simulink model "ADRClibriry"  (R2018a)
settings: Solver=VariableStepAuto  StartTime=0.0  StopTime=10.0  RelTol=1e-3
undefined symbols (not defined in the file or in its folder): sigbuilder_block
libraries: simulink x7, dspswit3 x4
(part 2 of 2)

== system ADRClibriry/ADRC_controller_NLSEF/roll_ADRC1 ==
  States : Inport  OutDataTypeStr=Bus: StatesBus
  <roll_cmd> : Inport  Port=2
  u_x : Inport  Port=3
  Bus Selector1 : BusSelector  OutputSignals=Euler
  ESO : Demux  Outputs=3
  Gain2 : Gain  Gain=0.025504
  Gain3 : Gain  Gain=39.2418
  MATLAB Function : MATLAB Function  TreatAsAtomicUnit=on
  Mux : Mux  Inputs=2
  RT : RateTransition  OutPortSampleTime=0.05
  RT1 : RateTransition  OutPortSampleTime=0.01
  S-Function : S-Function  FunctionName=s_TD  SFunctionDeploymentMode=off  EnableBusSupport=off
  S-Function4 : S-Function  FunctionName=s_ESO  SFunctionDeploymentMode=off  EnableBusSupport=off
  Scope : Scope  NumInputPorts=2
  Scope1 : Scope
  Scope2 : Scope  NumInputPorts=2
  Scope4 : Scope  NumInputPorts=2
  Sine Wave : Sin  Amplitude=0.2  Frequency=2*pi*1  Phase=2*pi*1.5  SampleTime=0.01
  TD : Demux  Outputs=2
  Terminator : Terminator
  Terminator1 : Terminator
  angle : Demux  Outputs=3
  "u_p " : Outport
  d_1 : Outport  Port=2
  wires:
  Mux/1 -> S-Function4/1
  States/1 -> Bus Selector1/1
  Gain3/1 -> Mux/2
  ESO/3 -> Gain2/1
  <roll_cmd>/1 -> RT/1, Scope/1
  angle/1 -> Scope2/2, Mux/1
  Bus Selector1/1 -> angle/1  "<Euler>"
  RT/1 -> S-Function/1
  S-Function4/1 -> ESO/1
  RT1/1 -> TD/1
  TD/2 -> MATLAB Function/2(x2_d), Scope1/1
  Gain2/1 -> d_1/1
  S-Function/1 -> RT1/1
  TD/1 -> MATLAB Function/1(x1_d), Scope/2
  angle/3 -> Terminator1/1
  angle/2 -> Terminator/1
  ESO/2 -> MATLAB Function/4(x2)
  MATLAB Function/1(y) -> "u_p "/1
  Sine Wave/1 -> Scope4/1
  ESO/1 -> MATLAB Function/3(x1), Scope2/1
  u_x/1 -> Gain3/1

== system ADRClibriry/ADRC_controller_NLSEF/yaw_ADRC ==
  States : Inport  OutDataTypeStr=Bus: StatesBus
  <yaw_cmd> : Inport  Port=2
  Add : Sum  Inputs=+-
  Bus Selector1 : BusSelector  OutputSignals=Euler
  Demux : Demux  Outputs=2
  ESO : Demux  Outputs=3
  Gain2 : Gain  Gain=0.00562
  Gain3 : Gain  Gain=1/0.00562
  MATLAB Function : MATLAB Function  TreatAsAtomicUnit=on
  Manual Switch : ManualSwitch  CurrentSetting=0
  Mux : Mux  Inputs=2
  RT : RateTransition
  RT1 : RateTransition
  S-Function : S-Function  FunctionName=s_yawTD  SFunctionDeploymentMode=off  EnableBusSupport=off
  S-Function4 : S-Function  FunctionName=s_ESO  SFunctionDeploymentMode=off  EnableBusSupport=off
  Scope{,1..2,4} (4 alike) : Scope  NumInputPorts=2
  Scope3 : Scope
  Sine Wave : Sin  Amplitude=0.05  Frequency=2*pi*1  SampleTime=0.01
  Terminator : Terminator
  Terminator1 : Terminator
  angle : Demux  Outputs=3
  u_r : Outport
  wires:
  Mux/1 -> S-Function4/1
  States/1 -> Bus Selector1/1
  ESO/1 -> Scope4/2, MATLAB Function/3(x1), Scope1/1
  Gain3/1 -> Mux/2
  ESO/3 -> Gain2/1
  <yaw_cmd>/1 -> Manual Switch/2, Scope/2
  ESO/2 -> MATLAB Function/4(x2)
  Bus Selector1/1 -> angle/1  "<Euler>"
  RT/1 -> S-Function/1
  S-Function4/1 -> ESO/1
  Add/1 -> Scope3/1, u_r/1, Gain3/1
  RT1/1 -> Demux/1
  Demux/2 -> Scope2/1, MATLAB Function/2(x2_d)
  Gain2/1 -> Add/2
  S-Function/1 -> RT1/1
  Demux/1 -> MATLAB Function/1(x1_d), Scope/1
  angle/3 -> Scope1/2, Mux/1
  angle/2 -> Terminator1/1
  angle/1 -> Terminator/1
  MATLAB Function/1(y) -> Add/1
  Sine Wave/1 -> Manual Switch/1, Scope4/1
  Manual Switch/1 -> RT/1

== system ADRClibriry/ADRC_controller_NLSEF1/Subsystem ==
  In1 : Inport
  In2 : Inport  Port=2
  In3 : Inport  Port=3
  Divide : Product  Inputs=*/
  Gain : Gain  Gain=-1225^2/9.788
  Product : Product
  Saturation1 : Saturate  UpperLimit=1  LowerLimit=0.5
  Sqrt : Sqrt  SaturateOnIntegerOverflow=on
  Trigonometric Function : Trigonometry  Operator=cos
  Trigonometric Function1 : Trigonometry  Operator=cos
  speed : Outport
  wires:
  Saturation1/1 -> Divide/2
  Trigonometric Function/1 -> Product/1
  In3/1 -> Divide/1
  Trigonometric Function1/1 -> Product/2
  In2/1 -> Trigonometric Function/1
  Product/1 -> Saturation1/1
  In1/1 -> Trigonometric Function1/1
  Divide/1 -> Gain/1
  Gain/1 -> Sqrt/1
  Sqrt/1 -> speed/1

== system ADRClibriry/ADRC_controller_NLSEF1/Subsystem2 ==
  u_1 : Inport
  u_2 : Inport  Port=2
  u_3 : Inport  Port=3
  u_4 : Inport  Port=4
  u_5 : Inport  Port=5
  d_3 : Inport  Port=6
  Demux3 : Demux  Outputs=7
  Mux : Mux  Inputs=6
  S-Function1 : S-Function  FunctionName=s_Optim1  SFunctionDeploymentMode=off  EnableBusSupport=off
  Saturation{1..4} (4 alike) : Saturate  UpperLimit=0.3491  LowerLimit=-0.3491
  c1 : Outport
  c2 : Outport  Port=2
  c3 : Outport  Port=3
  c4 : Outport  Port=4
  ux : Outport  Port=5
  uy : Outport  Port=6
  uz : Outport  Port=7
  wires:
  Demux3/4 -> Saturation4/1
  Saturation3/1 -> c3/1  "c3"
  u_3/1 -> Mux/3
  u_1/1 -> Mux/1
  Saturation1/1 -> c1/1  "c1"
  Demux3/1 -> Saturation1/1
  Saturation4/1 -> c4/1  "c4"
  Demux3/2 -> Saturation2/1
  u_2/1 -> Mux/2
  Saturation2/1 -> c2/1  "c2"
  Demux3/3 -> Saturation3/1
  Mux/1 -> S-Function1/1
  S-Function1/1 -> Demux3/1
  u_4/1 -> Mux/4
  d_3/1 -> Mux/6
  u_5/1 -> Mux/5
  Demux3/5 -> ux/1
  Demux3/6 -> uy/1
  Demux3/7 -> uz/1

== system ADRClibriry/ADRC_controller_NLSEF1/Subsystem3 ==
  u_p : Inport
  u_q : Inport  Port=2
  u_r : Inport  Port=3
  p : Inport  Port=4
  q : Inport  Port=5
  speed : Inport  Port=6
  Add1 : Sum
  Add2 : Sum  Inputs=+-
  Add3 : Sum  Inputs=+-
  Constant1 : Constant  Value=0.000029
  Constant2 : Constant  Value=0.04238
  Product{,1..3} (4 alike) : Product
  u_1 : Outport
  u_2 : Outport  Port=2
  u_3 : Outport  Port=3
  wires:
  Add3/1 -> u_3/1
  Add1/1 -> u_1/1
  Constant1/1 -> Product1/1, Product/2
  q/1 -> Product/1
  Product1/1 -> Product2/1
  Constant2/1 -> Add3/2
  u_p/1 -> Add1/2
  p/1 -> Product1/2
  Add2/1 -> u_2/1
  Product3/1 -> Add1/1
  speed/1 -> Product3/2, Product2/2
  Product/1 -> Product3/1
  Product2/1 -> Add2/2
  u_q/1 -> Add2/1
  u_r/1 -> Add3/1

== system ADRClibriry/ADRC_controller_NLSEF1/h_ADRC ==
  note: 控制器输出为升力提供的加速度
  States : Inport  OutDataTypeStr=Bus: StatesBus
  <throttle_cmd> : Inport  Port=2
  Add : Sum  Inputs=+-
  Bus Selector1 : BusSelector  OutputSignals=X_ned
  Constant : Constant  Value=9.78
  Demux : Demux  Outputs=2
  ESO : Demux  Outputs=3
  Gain2 : Gain
  Gain3 : Gain
  MATLAB Function : MATLAB Function  TreatAsAtomicUnit=on
  Mux : Mux  Inputs=2
  RT : RateTransition  OutPortSampleTime=0.05
  RT1 : RateTransition  OutPortSampleTime=0.01
  S-Function : S-Function  FunctionName=s_TD  SFunctionDeploymentMode=off  EnableBusSupport=off
  S-Function4 : S-Function  FunctionName=s_ESO  SFunctionDeploymentMode=off  EnableBusSupport=off
  Scope3 : Scope
  Sum2 : Sum  Inputs=++|
  Sum3 : Sum  Inputs=|++
  Terminator : Terminator
  Terminator1 : Terminator
  x : Demux  Outputs=3
  a_t : Outport
  wires:
  Mux/1 -> S-Function4/1
  States/1 -> Bus Selector1/1
  ESO/1 -> MATLAB Function/3(x1)
  Gain3/1 -> Sum2/2
  ESO/3 -> Sum3/1
  <throttle_cmd>/1 -> RT/1
  ESO/2 -> MATLAB Function/4(x2)
  Bus Selector1/1 -> x/1  "<X_ned>"
  RT/1 -> S-Function/1
  S-Function4/1 -> ESO/1
  RT1/1 -> Demux/1
  Demux/2 -> MATLAB Function/2(x2_d)
  Gain2/1 -> Add/2, Scope3/1
  S-Function/1 -> RT1/1
  Demux/1 -> MATLAB Function/1(x1_d)
  x/3 -> Mux/1
  x/2 -> Terminator/1
  x/1 -> Terminator1/1
  Add/1 -> a_t/1, Gain3/1  "a_t"
  Sum2/1 -> Mux/2
  Sum3/1 -> Gain2/1
  Constant/1 -> Sum3/2, Sum2/1
  MATLAB Function/1(y) -> Add/1

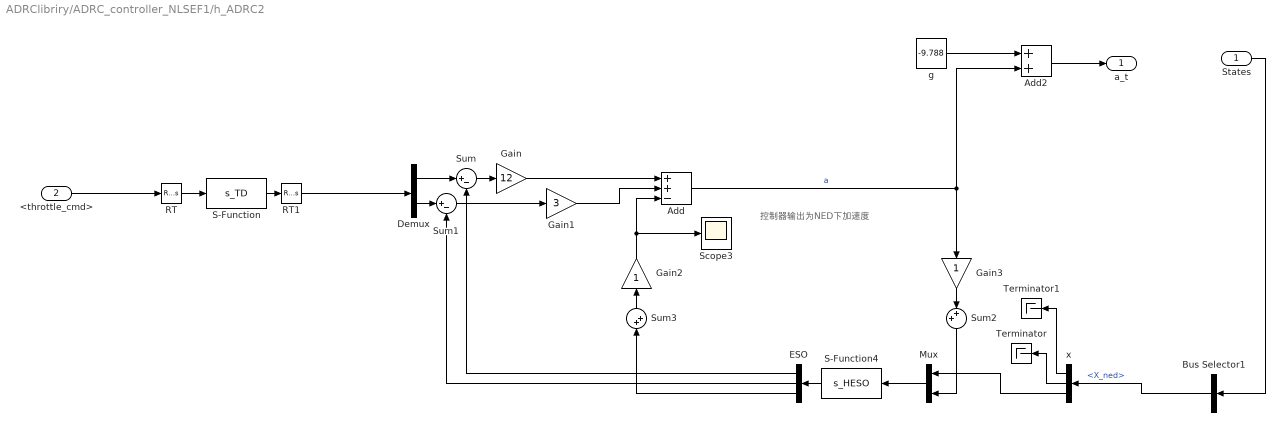
== system ADRClibriry/ADRC_controller_NLSEF1/h_ADRC2 ==
  note: 控制器输出为NED下加速度
  States : Inport  OutDataTypeStr=Bus: StatesBus
  <throttle_cmd> : Inport  Port=2
  Add : Sum  Inputs=++-
  Add2 : Sum
  Bus Selector1 : BusSelector  OutputSignals=X_ned
  Demux : Demux  Outputs=2
  ESO : Demux  Outputs=3
  Gain : Gain  Gain=12
  Gain1 : Gain  Gain=3
  Gain2 : Gain
  Gain3 : Gain
  Mux : Mux  Inputs=2
  RT : RateTransition  OutPortSampleTime=0.05
  RT1 : RateTransition  OutPortSampleTime=0.01
  S-Function : S-Function  FunctionName=s_TD  SFunctionDeploymentMode=off  EnableBusSupport=off
  S-Function4 : S-Function  FunctionName=s_HESO  SFunctionDeploymentMode=off  EnableBusSupport=off
  Scope3 : Scope
  Sum : Sum  Inputs=|+-
  Sum1 : Sum  Inputs=|+-
  Sum2 : Sum  Inputs=++|
  Sum3 : Sum  Inputs=|++
  Terminator : Terminator
  Terminator1 : Terminator
  g : Constant  Value=-9.788
  x : Demux  Outputs=3
  a_t : Outport
  wires:
  Gain1/1 -> Add/2
  Mux/1 -> S-Function4/1
  States/1 -> Bus Selector1/1
  ESO/1 -> Sum/2
  Gain3/1 -> Sum2/2
  ESO/3 -> Sum3/1
  <throttle_cmd>/1 -> RT/1
  ESO/2 -> Sum1/2
  Bus Selector1/1 -> x/1  "<X_ned>"
  RT/1 -> S-Function/1
  S-Function4/1 -> ESO/1
  Sum1/1 -> Gain1/1
  Gain/1 -> Add/1
  RT1/1 -> Demux/1
  Demux/2 -> Sum1/1
  Gain2/1 -> Add/3, Scope3/1
  S-Function/1 -> RT1/1
  Sum/1 -> Gain/1
  Demux/1 -> Sum/1
  x/3 -> Mux/1
  x/2 -> Terminator/1
  x/1 -> Terminator1/1
  Add/1 -> Add2/2, Gain3/1  "a"
  Sum2/1 -> Mux/2
  Sum3/1 -> Gain2/1
  Add2/1 -> a_t/1
  g/1 -> Add2/1

== system ADRClibriry/ADRC_controller_NLSEF1/h_ADRC3 ==
  note: 控制器输出为升力
  States : Inport  OutDataTypeStr=Bus: StatesBus
  <throttle_cmd> : Inport  Port=2
  Add : Sum  Inputs=++-
  Bus Selector1 : BusSelector  OutputSignals=X_ned
  Constant : Constant  Value=9.78
  Demux : Demux  Outputs=2
  ESO : Demux  Outputs=3
  Gain : Gain  Gain=12
  Gain1 : Gain  Gain=3
  Gain2 : Gain  Gain=1.53
  Gain3 : Gain  Gain=1/1.53
  Gain4 : Gain  Gain=1/1.53
  Mux : Mux  Inputs=2
  RT : RateTransition  OutPortSampleTime=0.05
  RT1 : RateTransition  OutPortSampleTime=0.01
  S-Function : S-Function  FunctionName=s_TD  SFunctionDeploymentMode=off  EnableBusSupport=off
  S-Function4 : S-Function  FunctionName=s_HESO  SFunctionDeploymentMode=off  EnableBusSupport=off
  Sum : Sum  Inputs=|+-
  Sum1 : Sum  Inputs=|+-
  Sum2 : Sum  Inputs=++|
  Sum3 : Sum  Inputs=|++
  Terminator : Terminator
  Terminator1 : Terminator
  x : Demux  Outputs=3
  a_t : Outport
  wires:
  Gain1/1 -> Add/2
  Mux/1 -> S-Function4/1
  States/1 -> Bus Selector1/1
  ESO/1 -> Sum/2
  Gain3/1 -> Sum2/2
  ESO/3 -> Sum3/1
  <throttle_cmd>/1 -> RT/1
  ESO/2 -> Sum1/2
  Bus Selector1/1 -> x/1  "<X_ned>"
  RT/1 -> S-Function/1
  S-Function4/1 -> ESO/1
  Sum1/1 -> Gain1/1
  Gain/1 -> Add/1
  RT1/1 -> Demux/1
  Demux/2 -> Sum1/1
  Gain2/1 -> Add/3
  S-Function/1 -> RT1/1
  Sum/1 -> Gain/1
  Demux/1 -> Sum/1
  x/3 -> Mux/1
  x/2 -> Terminator/1
  x/1 -> Terminator1/1
  Add/1 -> Gain4/1, Gain3/1  "T"
  Sum2/1 -> Mux/2
  Sum3/1 -> Gain2/1
  Constant/1 -> Sum3/2, Sum2/1
  Gain4/1 -> a_t/1

== system ADRClibriry/ADRC_controller_NLSEF1/pitch_ADRC ==
  States : Inport  OutDataTypeStr=Bus: StatesBus
  <pitch_cmd> : Inport  Port=2
  u_y : Inport  Port=3
  Add : Sum  Inputs=+-
  Bus Selector1 : BusSelector  OutputSignals=Euler
  Demux : Demux  Outputs=2
  ESO : Demux  Outputs=3
  Gain : Gain  Gain=0.025504
  Gain5 : Gain  Gain=39.2418
  MATLAB Function : MATLAB Function  TreatAsAtomicUnit=on
  Mux : Mux  Inputs=2
  RT : RateTransition  OutPortSampleTime=0.05
  RT1 : RateTransition  OutPortSampleTime=0.01
  S-Function : S-Function  FunctionName=s_TD  SFunctionDeploymentMode=off  EnableBusSupport=off
  S-Function4 : S-Function  FunctionName=s_ESO  SFunctionDeploymentMode=off  EnableBusSupport=off
  Scope4 : Scope  NumInputPorts=2
  Sine Wave : Sin  Amplitude=0.2  Frequency=2*pi*1  SampleTime=0.01
  Terminator : Terminator
  Terminator1 : Terminator
  angle : Demux  Outputs=3
  "u_q " : Outport
  wires:
  Mux/1 -> S-Function4/1
  States/1 -> Bus Selector1/1
  Gain5/1 -> Mux/2
  ESO/3 -> Gain/1
  Bus Selector1/1 -> angle/1  "<Euler>"
  RT/1 -> S-Function/1
  S-Function4/1 -> ESO/1
  RT1/1 -> Demux/1
  Demux/2 -> MATLAB Function/2(x2_d)
  S-Function/1 -> RT1/1
  angle/3 -> Terminator1/1
  angle/2 -> Mux/1
  ESO/2 -> MATLAB Function/4(x2)
  Demux/1 -> MATLAB Function/1(x1_d)
  <pitch_cmd>/1 -> RT/1
  angle/1 -> Terminator/1
  ESO/1 -> MATLAB Function/3(x1)
  Sine Wave/1 -> Scope4/1
  MATLAB Function/1(y) -> Add/1
  Add/1 -> "u_q "/1
  u_y/1 -> Gain5/1
  Gain/1 -> Add/2

== system ADRClibriry/ADRC_controller_NLSEF1/roll_ADRC ==
  States : Inport  OutDataTypeStr=Bus: StatesBus
  <roll_cmd> : Inport  Port=2
  u_x : Inport  Port=3
  Add : Sum  Inputs=+-
  Bus Selector1 : BusSelector  OutputSignals=Euler
  ESO : Demux  Outputs=3
  Gain2 : Gain  Gain=0.025504
  Gain3 : Gain  Gain=39.2418
  MATLAB Function : MATLAB Function  TreatAsAtomicUnit=on
  Mux : Mux  Inputs=2
  RT : RateTransition  OutPortSampleTime=0.05
  RT1 : RateTransition  OutPortSampleTime=0.01
  S-Function : S-Function  FunctionName=s_TD  SFunctionDeploymentMode=off  EnableBusSupport=off
  S-Function4 : S-Function  FunctionName=s_ESO  SFunctionDeploymentMode=off  EnableBusSupport=off
  Scope : Scope  NumInputPorts=2
  Scope1 : Scope
  Scope2 : Scope  NumInputPorts=2
  Scope4 : Scope  NumInputPorts=2
  Sine Wave : Sin  Amplitude=0.2  Frequency=2*pi*1  Phase=2*pi*1.5  SampleTime=0.01
  TD : Demux  Outputs=2
  Terminator : Terminator
  Terminator1 : Terminator
  angle : Demux  Outputs=3
  "u_p " : Outport
  wires:
  RT/1 -> S-Function/1
  ESO/3 -> Gain2/1
  S-Function4/1 -> ESO/1
  RT1/1 -> TD/1
  angle/2 -> Terminator/1
  Gain2/1 -> Add/2
  MATLAB Function/1(y) -> Add/1
  angle/1 -> Scope2/2, Mux/1
  Bus Selector1/1 -> angle/1  "<Euler>"
  Sine Wave/1 -> Scope4/1
  TD/2 -> MATLAB Function/2(x2_d), Scope1/1
  ESO/2 -> MATLAB Function/4(x2)
  Gain3/1 -> Mux/2
  S-Function/1 -> RT1/1
  ESO/1 -> MATLAB Function/3(x1), Scope2/1
  States/1 -> Bus Selector1/1
  Mux/1 -> S-Function4/1
  TD/1 -> MATLAB Function/1(x1_d), Scope/2
  u_x/1 -> Gain3/1
  angle/3 -> Terminator1/1
  <roll_cmd>/1 -> RT/1, Scope/1
  Add/1 -> "u_p "/1

== system ADRClibriry/ADRC_controller_NLSEF1/roll_ADRC1 ==
  States : Inport  OutDataTypeStr=Bus: StatesBus
  <roll_cmd> : Inport  Port=2
  u_x : Inport  Port=3
  Bus Selector1 : BusSelector  OutputSignals=Euler
  ESO : Demux  Outputs=3
  Gain2 : Gain  Gain=0.025504
  Gain3 : Gain  Gain=39.2418
  MATLAB Function : MATLAB Function  TreatAsAtomicUnit=on
  Mux : Mux  Inputs=2
  RT : RateTransition  OutPortSampleTime=0.05
  RT1 : RateTransition  OutPortSampleTime=0.01
  S-Function : S-Function  FunctionName=s_TD  SFunctionDeploymentMode=off  EnableBusSupport=off
  S-Function4 : S-Function  FunctionName=s_ESO  SFunctionDeploymentMode=off  EnableBusSupport=off
  Scope : Scope  NumInputPorts=2
  Scope1 : Scope
  Scope2 : Scope  NumInputPorts=2
  Scope4 : Scope  NumInputPorts=2
  Sine Wave : Sin  Amplitude=0.2  Frequency=2*pi*1  Phase=2*pi*1.5  SampleTime=0.01
  TD : Demux  Outputs=2
  Terminator : Terminator
  Terminator1 : Terminator
  angle : Demux  Outputs=3
  "u_p " : Outport
  d_1 : Outport  Port=2
  wires:
  Mux/1 -> S-Function4/1
  States/1 -> Bus Selector1/1
  Gain3/1 -> Mux/2
  ESO/3 -> Gain2/1
  <roll_cmd>/1 -> RT/1, Scope/1
  angle/1 -> Scope2/2, Mux/1
  Bus Selector1/1 -> angle/1  "<Euler>"
  RT/1 -> S-Function/1
  S-Function4/1 -> ESO/1
  RT1/1 -> TD/1
  TD/2 -> MATLAB Function/2(x2_d), Scope1/1
  Gain2/1 -> d_1/1
  S-Function/1 -> RT1/1
  TD/1 -> MATLAB Function/1(x1_d), Scope/2
  angle/3 -> Terminator1/1
  angle/2 -> Terminator/1
  ESO/2 -> MATLAB Function/4(x2)
  MATLAB Function/1(y) -> "u_p "/1
  Sine Wave/1 -> Scope4/1
  ESO/1 -> MATLAB Function/3(x1), Scope2/1
  u_x/1 -> Gain3/1

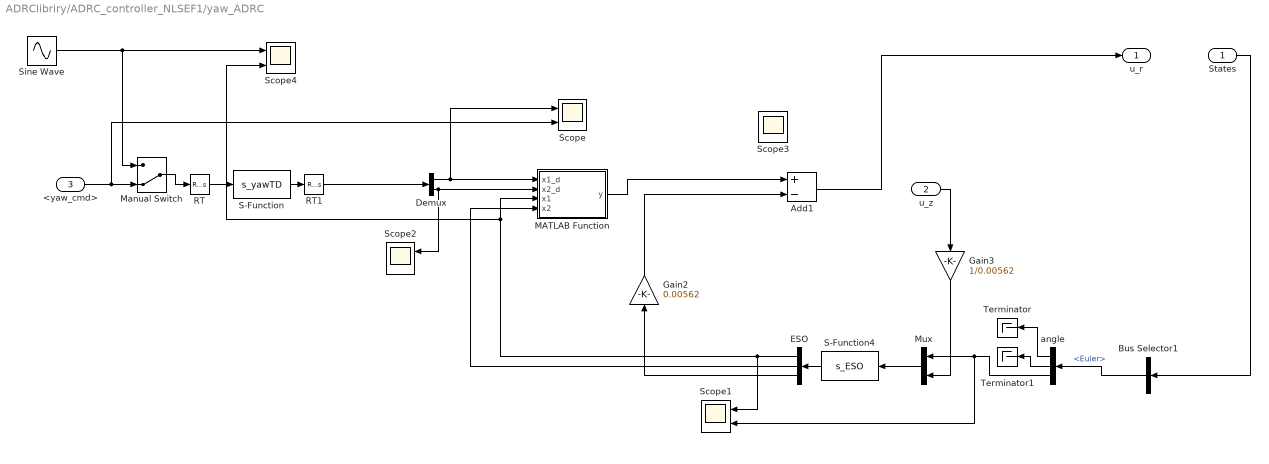
== system ADRClibriry/ADRC_controller_NLSEF1/yaw_ADRC ==
  States : Inport  OutDataTypeStr=Bus: StatesBus
  u_z : Inport  Port=2
  <yaw_cmd> : Inport  Port=3
  Add1 : Sum  Inputs=+-
  Bus Selector1 : BusSelector  OutputSignals=Euler
  Demux : Demux  Outputs=2
  ESO : Demux  Outputs=3
  Gain2 : Gain  Gain=0.00562
  Gain3 : Gain  Gain=1/0.00562
  MATLAB Function : MATLAB Function  TreatAsAtomicUnit=on
  Manual Switch : ManualSwitch  CurrentSetting=0
  Mux : Mux  Inputs=2
  RT : RateTransition
  RT1 : RateTransition
  S-Function : S-Function  FunctionName=s_yawTD  SFunctionDeploymentMode=off  EnableBusSupport=off
  S-Function4 : S-Function  FunctionName=s_ESO  SFunctionDeploymentMode=off  EnableBusSupport=off
  Scope{,1..2,4} (4 alike) : Scope  NumInputPorts=2
  Scope3 : Scope
  Sine Wave : Sin  Amplitude=0.05  Frequency=2*pi*1  SampleTime=0.01
  Terminator : Terminator
  Terminator1 : Terminator
  angle : Demux  Outputs=3
  u_r : Outport
  wires:
  Mux/1 -> S-Function4/1
  States/1 -> Bus Selector1/1
  ESO/1 -> Scope4/2, MATLAB Function/3(x1), Scope1/1
  Gain3/1 -> Mux/2
  ESO/3 -> Gain2/1
  <yaw_cmd>/1 -> Manual Switch/2, Scope/2
  ESO/2 -> MATLAB Function/4(x2)
  Bus Selector1/1 -> angle/1  "<Euler>"
  RT/1 -> S-Function/1
  S-Function4/1 -> ESO/1
  RT1/1 -> Demux/1
  Demux/2 -> Scope2/1, MATLAB Function/2(x2_d)
  S-Function/1 -> RT1/1
  Demux/1 -> MATLAB Function/1(x1_d), Scope/1
  angle/3 -> Scope1/2, Mux/1
  angle/2 -> Terminator1/1
  angle/1 -> Terminator/1
  Sine Wave/1 -> Manual Switch/1, Scope4/1
  Manual Switch/1 -> RT/1
  Gain2/1 -> Add1/2
  MATLAB Function/1(y) -> Add1/1
  Add1/1 -> u_r/1
  u_z/1 -> Gain3/1

== system ADRClibriry/PID_controller1/Signal Builder ==
  Demux : Demux  Tag=STV Demux
  FromWs : FromWorkspace  Tag=STV FromWs  VariableName=tuvar  SampleTime=0
      SigBuilderData=|
      | common.afterFinalStr = 'Extrapolate'
      | common.sampleTime = 0
      | dataSet.timeRange = [0 50]
      | dataSet.name = 'Group 1'
      | sbobj.Groups.Name = 'Group 1'
      | sbobj.Groups.Signals(1).Name = 'roll_cmd'
      | sbobj.Groups.Signals(1).XData = [0 6 6 8.55 8.55 10.7 10.7 13 13 50]
      | sbobj.Groups.Signals(1).YData = [0 0 0.05 0.05 0 0 -0.05 -0.05 0 0]
      | sbobj.Groups.Signals(2).Name = 'picth_cmd'
      | sbobj.Groups.Signals(2).XData = [0 14.9 14.9 17.5 17.5 20.8 50]
      | sbobj.Groups.Signals(2).YData = [0 0 0.05 0.05 0 0 0]
      | sbobj.Groups.Signals(3).Name = 'yaw_cmd'
      | sbobj.Groups.Signals(3).XData = [0 33.4 33.4 39.4 39.4 40.9 40.9 46.65 46.65 50]
      | sbobj.Groups.Signals(3).YData = [0 0 0.1 0.1 0 0 -0.1 -0.1 0 0]
      | sbobj.Groups.Signals(4).Name = 'throttle_cmd'
      | sbobj.Groups.Signals(4).XData = [0 10 21.35 21.35 26.15 32.4 50]
      | sbobj.Groups.Signals(4).YData = [0 -1.8 -1.8 -3.8 -3.8 -3.8 -3.8]
      | sbobj.Groups.TimeRange = [0 50]
  roll_cmd : Outport  Tag=STV Outport
  picth_cmd : Outport  Tag=STV Outport  Port=2
  yaw_cmd : Outport  Tag=STV Outport  Port=3
  throttle_cmd : Outport  Tag=STV Outport  Port=4
  wires:
  Demux/1 -> roll_cmd/1
  FromWs/1 -> Demux/1
  Demux/2 -> picth_cmd/1
  Demux/3 -> yaw_cmd/1
  Demux/4 -> throttle_cmd/1

== system ADRClibriry/PID_controller1/Subsystem ==
  In1 : Inport
  In2 : Inport  Port=2
  In3 : Inport  Port=3
  Divide : Product  Inputs=*/
  Gain : Gain  Gain=-1225^2/9.788
  Product : Product
  Saturation1 : Saturate  UpperLimit=1  LowerLimit=0.5
  Sqrt : Sqrt  SaturateOnIntegerOverflow=on
  Trigonometric Function : Trigonometry  Operator=cos
  Trigonometric Function1 : Trigonometry  Operator=cos
  speed : Outport
  wires:
  Saturation1/1 -> Divide/2
  Trigonometric Function/1 -> Product/1
  In3/1 -> Divide/1
  Trigonometric Function1/1 -> Product/2
  In2/1 -> Trigonometric Function/1
  Product/1 -> Saturation1/1
  In1/1 -> Trigonometric Function1/1
  Divide/1 -> Gain/1
  Gain/1 -> Sqrt/1
  Sqrt/1 -> speed/1

== system ADRClibriry/PID_controller1/Subsystem2 ==
  u_1 : Inport
  u_2 : Inport  Port=2
  u_3 : Inport  Port=3
  u_4 : Inport  Port=4
  u_5 : Inport  Port=5
  d_3 : Inport  Port=6
  Demux3 : Demux  Outputs=7
  Mux : Mux  Inputs=6
  S-Function1 : S-Function  FunctionName=s_Optim2  SFunctionDeploymentMode=off  EnableBusSupport=off
  Saturation{1..4} (4 alike) : Saturate  UpperLimit=0.3491  LowerLimit=-0.3491
  c1 : Outport
  c2 : Outport  Port=2
  c3 : Outport  Port=3
  c4 : Outport  Port=4
  ux : Outport  Port=5
  uy : Outport  Port=6
  uz : Outport  Port=7
  wires:
  Demux3/4 -> Saturation4/1
  Saturation3/1 -> c3/1  "c3"
  u_3/1 -> Mux/3
  u_1/1 -> Mux/1
  Saturation1/1 -> c1/1  "c1"
  Demux3/1 -> Saturation1/1
  Saturation4/1 -> c4/1  "c4"
  Demux3/2 -> Saturation2/1
  u_2/1 -> Mux/2
  Saturation2/1 -> c2/1  "c2"
  Demux3/3 -> Saturation3/1
  Mux/1 -> S-Function1/1
  S-Function1/1 -> Demux3/1
  u_4/1 -> Mux/4
  d_3/1 -> Mux/6
  u_5/1 -> Mux/5
  Demux3/5 -> ux/1
  Demux3/6 -> uy/1
  Demux3/7 -> uz/1

== system ADRClibriry/PID_controller1/Subsystem3 ==
  u_p : Inport
  p : Inport  Port=2
  u_q : Inport  Port=3
  q : Inport  Port=4
  u_r : Inport  Port=5
  speed : Inport  Port=6
  Add1 : Sum
  Add2 : Sum  Inputs=+-
  Add3 : Sum  Inputs=+-
  Constant1 : Constant  Value=0.000029
  Constant2 : Constant  Value=0.04238
  Product{,1..3} (4 alike) : Product
  u_1 : Outport
  u_2 : Outport  Port=2
  u_3 : Outport  Port=3
  wires:
  Add3/1 -> u_3/1
  Add1/1 -> u_1/1
  Constant1/1 -> Product1/1, Product/2
  q/1 -> Product/1
  Product1/1 -> Product2/1
  Constant2/1 -> Add3/2
  u_p/1 -> Add1/2
  p/1 -> Product1/2
  Add2/1 -> u_2/1
  Product3/1 -> Add1/1
  speed/1 -> Product3/2, Product2/2
  Product/1 -> Product3/1
  Product2/1 -> Add2/2
  u_q/1 -> Add2/1
  u_r/1 -> Add3/1

== matlab function ADRClibriry/ADRC_controller_NLSEF/MATLAB Function ==
  data: u input; y output
function y = fcn(u)
K=1*[-0.56   0       0.56    0;
          0  -0.56    0       0.56;
      0.218   0.218   0.218   0.218];
 M=K*u;
y = M(1);

== matlab function ADRClibriry/ADRC_controller_LSEF/Subsystem2/MATLAB Function ==
  data: u input; y output
function y = Torque2surface(u)
A=0.349;
u_1=u(1);
u_2=u(2);
u_3=u(3);
yaw_allowance=[0;0;0];
d=[0;0];
yaw_allowance(1)=A-abs(u_1);
yaw_allowance(2)=A-abs(u_2);
yaw_allowance(3)=2*(yaw_allowance(1)+yaw_allowance(2));    
yaw_sign=sign(u_3);
if  yaw_allowance(1)<yaw_allowance(2)   
    if abs(u_3)<2*yaw_allowance(1)   
        d(1)=0.5*u_3;
        d(2)=0.5*u_3;   
    elseif abs(u_3)>yaw_allowance(3)  
        d(1)=yaw_sign*yaw_allowance(1);
        d(2)=yaw_sign*yaw_allowance(2);   
    else  
        d(1)=yaw_sign*yaw_allowance(1);
        d(2)=yaw_sign*(abs(u_3)-yaw_allowance(1));
    end
else
    if abs(u_3)<2*yaw_allowance(2)   
        d(1)=0.5*u_3;
        d(2)=0.5*u_3; 
    elseif abs(u_3)>yaw_allowance(3)
        d(1)=yaw_sign*yaw_allowance(1);
        d(2)=yaw_sign*yaw_allowance(2);  
    else
        d(1)=yaw_sign*(abs(u_3)-yaw_allowance(2));
        d(2)=yaw_sign*yaw_allowance(2);
    end
end
c1=-u_1+d(1);
c2=-u_2+d(2);
c3= u_1+d(1);
c4= u_2+d(2);
y = [c1;c2;c3;c4];

== matlab function ADRClibriry/ADRC_controller_NLSEF/MATLAB Function1 ==
  data: u input; y output
function y = fcn(u)
K=1*[-0.56   0       0.56    0;
          0  -0.56    0       0.56;
      0.218   0.218   0.218   0.218];
 M=K*u;
y = M(2);

== matlab function ADRClibriry/ADRC_controller_NLSEF/MATLAB Function2 ==
  data: u input; y output
function y = fcn(u)
K=1*[-0.56   0       0.56    0;
          0  -0.56    0       0.56;
      0.218   0.218   0.218   0.218];
 M=K*u;
y = M(3);

== matlab function ADRClibriry/ADRC_controller_NLSEF/Subsystem2/MATLAB Function ==
  data: u input; y output
function y = Torque2surface(u)
A=0.349;
u_1=u(1);
u_2=u(2);
u_3=u(3);
yaw_allowance=[0;0;0];
d=[0;0];
yaw_allowance(1)=A-abs(u_1);
yaw_allowance(2)=A-abs(u_2);
yaw_allowance(3)=2*(yaw_allowance(1)+yaw_allowance(2));    
yaw_sign=sign(u_3);
if  yaw_allowance(1)<yaw_allowance(2)   
    if abs(u_3)<2*yaw_allowance(1)   
        d(1)=0.5*u_3;
        d(2)=0.5*u_3;   
    elseif abs(u_3)>yaw_allowance(3)  
        d(1)=yaw_sign*yaw_allowance(1);
        d(2)=yaw_sign*yaw_allowance(2);   
    else  
        d(1)=yaw_sign*yaw_allowance(1);
        d(2)=yaw_sign*(abs(u_3)-yaw_allowance(1));
    end
else
    if abs(u_3)<2*yaw_allowance(2)   
        d(1)=0.5*u_3;
        d(2)=0.5*u_3; 
    elseif abs(u_3)>yaw_allowance(3)
        d(1)=yaw_sign*yaw_allowance(1);
        d(2)=yaw_sign*yaw_allowance(2);  
    else
        d(1)=yaw_sign*(abs(u_3)-yaw_allowance(2));
        d(2)=yaw_sign*yaw_allowance(2);
    end
end
c1=-u_1+d(1);
c2=-u_2+d(2);
c3= u_1+d(1);
c4= u_2+d(2);
y = [c1;c2;c3;c4];

== matlab function ADRClibriry/ADRC_controller_NLSEF/pitch_ADRC/MATLAB Function ==
  data: x1_d input; y output; x2_d input; x1 input; x2 input
function y = NLSEF_pitch(x1_d,x2_d,x1,x2)
e1=x1_d-x1;
e2=x2_d-x2;
kp=1;kd=1.3;
alfa1=0.75;alfa2=1.5;
delta=0.1;
y = kp*fal(e1,alfa1,delta)+kd*fal(e2,alfa2,delta);   % 控制输出
end

== matlab function ADRClibriry/ADRC_controller_NLSEF/roll_ADRC/MATLAB Function ==
  data: x1_d input; y output; x2_d input; x1 input; x2 input
function y = NLSEF_roll(x1_d,x2_d,x1,x2)
e1=x1_d-x1;
e2=x2_d-x2;
kp=1;kd=1.3;
alfa1=0.75;alfa2=1.5;
delta=0.1;
y = kp*fal(e1,alfa1,delta)+kd*fal(e2,alfa2,delta);   % 控制输出
end

== matlab function ADRClibriry/ADRC_controller_NLSEF/yaw_ADRC/MATLAB Function ==
  data: x1_d input; y output; x2_d input; x1 input; x2 input
function y = NLSEF_yaw(x1_d,x2_d,x1,x2)
e1=x1_d-x1;
e2=x2_d-x2;
kp=1;kd=0.5;
alfa1=0.75;alfa2=1.5;
delta=0.1;
y = kp*fal(e1,alfa1,delta)+kd*fal(e2,alfa2,delta);  
end

== matlab function ADRClibriry/ADRC_controller_NLSEF/h_ADRC/MATLAB Function ==
  data: x1_d input; y output; x2_d input; x1 input; x2 input
function y = NLSEF_H(x1_d,x2_d,x1,x2)
e1=x1_d-x1;
e2=x2_d-x2;
kp=3;kd=2;
alfa1=0.75;alfa2=1.5;
delta=0.1;
y = kp*fal(e1,alfa1,delta)+kd*fal(e2,alfa2,delta);

== matlab function ADRClibriry/ADRC_controller_NLSEF/roll_ADRC1/MATLAB Function ==
  data: x1_d input; y output; x2_d input; x1 input; x2 input
function y = NLSEF_roll(x1_d,x2_d,x1,x2)
e1=x1_d-x1;
e2=x2_d-x2;
kp=1;kd=1.3;
alfa1=0.75;alfa2=1.5;
delta=0.1;
y = kp*fal(e1,alfa1,delta)+kd*fal(e2,alfa2,delta);   % 控制输出
end

== matlab function ADRClibriry/ADRC_controller_NLSEF1/h_ADRC/MATLAB Function ==
  data: x1_d input; y output; x2_d input; x1 input; x2 input
function y = NLSEF_H(x1_d,x2_d,x1,x2)
e1=x1_d-x1;
e2=x2_d-x2;
kp=3;kd=2;
alfa1=0.75;alfa2=1.5;
delta=0.1;
y = kp*fal(e1,alfa1,delta)+kd*fal(e2,alfa2,delta);

== matlab function ADRClibriry/ADRC_controller_NLSEF1/pitch_ADRC/MATLAB Function ==
  data: x1_d input; y output; x2_d input; x1 input; x2 input
function y = NLSEF_pitch(x1_d,x2_d,x1,x2)
e1=x1_d-x1;
e2=x2_d-x2;
kp=1;kd=1.3;
alfa1=0.75;alfa2=1.5;
delta=0.1;
y = kp*fal(e1,alfa1,delta)+kd*fal(e2,alfa2,delta);   % 控制输出
end

== matlab function ADRClibriry/ADRC_controller_NLSEF1/roll_ADRC/MATLAB Function ==
  data: x1_d input; y output; x2_d input; x1 input; x2 input
function y = NLSEF_roll(x1_d,x2_d,x1,x2)
e1=x1_d-x1;
e2=x2_d-x2;
kp=1;kd=1.3;
alfa1=0.75;alfa2=1.5;
delta=0.1;
y = kp*fal(e1,alfa1,delta)+kd*fal(e2,alfa2,delta);   % 控制输出
end

== matlab function ADRClibriry/ADRC_controller_NLSEF1/roll_ADRC1/MATLAB Function ==
  data: x1_d input; y output; x2_d input; x1 input; x2 input
function y = NLSEF_roll(x1_d,x2_d,x1,x2)
e1=x1_d-x1;
e2=x2_d-x2;
kp=1;kd=1.3;
alfa1=0.75;alfa2=1.5;
delta=0.1;
y = kp*fal(e1,alfa1,delta)+kd*fal(e2,alfa2,delta);   % 控制输出
end

== matlab function ADRClibriry/ADRC_controller_NLSEF1/yaw_ADRC/MATLAB Function ==
  data: x1_d input; y output; x2_d input; x1 input; x2 input
function y = NLSEF_yaw(x1_d,x2_d,x1,x2)
e1=x1_d-x1;
e2=x2_d-x2;
kp=1;kd=0.5;
alfa1=0.75;alfa2=1.5;
delta=0.1;
y = kp*fal(e1,alfa1,delta)+kd*fal(e2,alfa2,delta);  
end

== matlab function ADRClibriry/PID_controller1/MATLAB Function ==
  data: u input; y output
function y = Eulerrate2pqr(u)
Roll=u(4);
Pitch=u(5);
Q=[1    sin(Roll)*tan(Pitch)    cos(Roll)*tan(Pitch);
   0        cos(Roll)               -sin(Roll);
   0    sin(Roll)*sec(Pitch)    cos(Roll)*sec(Pitch)];
y = Q\[u(1);u(2);u(3)];

== matlab function ADRClibriry/PID_controller1/MATLAB Function1 ==
  data: u input; y output
function y = Yawcontrol(u)
if u<-pi
    a=u+2*pi;
elseif u>=pi
    a=u-2*pi;
else   
    a=u;
end
y = a;
